simulink model "linear"  (R2019a)
settings: Solver=VariableStepAuto  StartTime=0.0  StopTime=1500  RelTol=1e-3
settings Model: Creator=josefernandorosaribeiro  LastModifiedBy=josefernandorosaribeiro

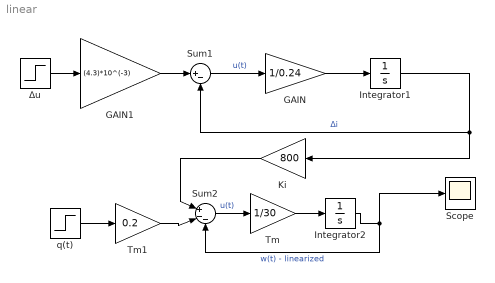
== system linear ==
  GAIN : Gain  Gain=1/0.24
  GAIN1 : Gain  Gain=(4.3)*10^(-3)
  Integrator1 : Integrator  InitialCondition=0.0072
  Integrator2 : Integrator  InitialCondition=0.0072
  Ki : Gain  Gain=800
  Scope : Scope
  Sum1 : Sum  Inputs=|+-
  Sum2 : Sum  Inputs=|+--
  Tm : Gain  Gain=1/30
  Tm1 : Gain  Gain=0.2
  q(t) : Step  Before=5  After=5  SampleTime=0
  Δu : Step  Before=1  After=5  SampleTime=0
  wires:
  Δu/1 -> GAIN1/1
  Integrator1/1 -> Sum1/2, Ki/1  "Δi"
  Sum1/1 -> GAIN/1  "u(t)"
  GAIN/1 -> Integrator1/1
  Tm/1 -> Integrator2/1
  Sum2/1 -> Tm/1  "u(t)"
  Ki/1 -> Sum2/1
  Tm1/1 -> Sum2/2
  q(t)/1 -> Tm1/1
  GAIN1/1 -> Sum1/1
  Integrator2/1 -> Scope/1, Sum2/3  "w(t) - linearized"
